simulink model "Task4Lab7Cs"  (R2015a)
settings: Solver=ode45  StartTime=0.0  StopTime=70  RelTol=1e-3
settings Model: Creator=Quswar Mahmood Abid  LastModifiedBy=Quswar Mahmood Abid

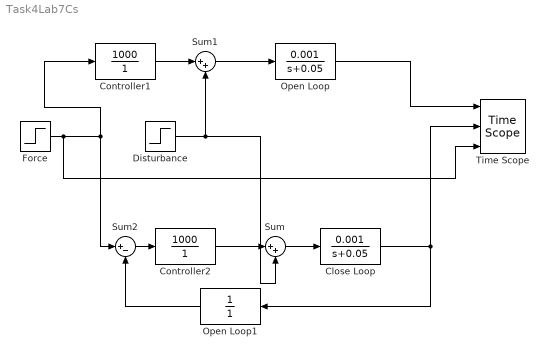
== system Task4Lab7Cs ==
  Close Loop : TransferFcn  Numerator=[0.001]  Denominator=[1 0.05]
  Controller1 : TransferFcn  Numerator=[1000]  Denominator=[1]
  Controller2 : TransferFcn  Numerator=[1000]  Denominator=[1]
  Disturbance : Step  Time=0  After=5000  SampleTime=0
  Force : Step  Time=0  After=500  SampleTime=0
  Open Loop : TransferFcn  Numerator=[0.001]  Denominator=[1 0.05]
  Open Loop1 : TransferFcn  Denominator=[1]
  Sum : Sum  Inputs=|++
  Sum1 : Sum  Inputs=|++
  Sum2 : Sum  Inputs=|+-
  Time Scope : TimeScope  DefaultConfigurationName=spbscopes.TimeScopeBlockCfg  NumInputPorts=3
  wires:
  Disturbance/1 -> Sum/2, Sum1/2
  Force/1 -> Time Scope/3, Controller1/1, Sum2/1
  Sum1/1 -> Open Loop/1
  Open Loop1/1 -> Sum2/2
  Controller1/1 -> Sum1/1
  Open Loop/1 -> Time Scope/1
  Sum2/1 -> Controller2/1
  Controller2/1 -> Sum/1
  Sum/1 -> Close Loop/1
  Close Loop/1 -> Open Loop1/1, Time Scope/2
